simulink model "SIR"  (R2024b)
settings: Solver=VariableStepAuto  StartTime=0.0  StopTime=50.0  RelTol=1e-3
settings Model: Creator=max  LastModifiedBy=max

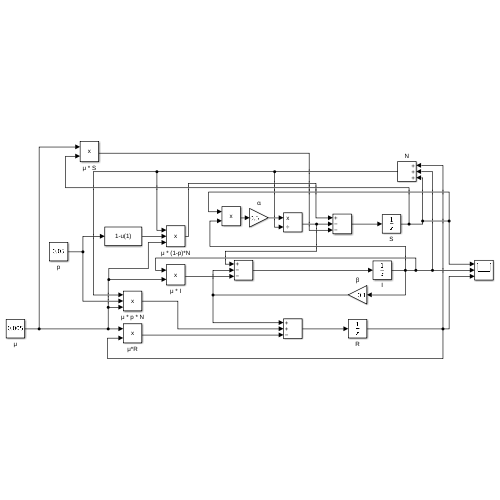
[thumbnail: Simulink's stored preview of the top-level diagram]
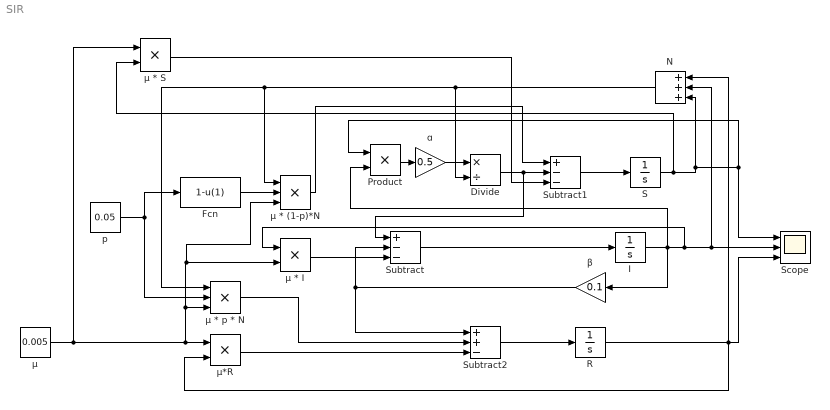
== system SIR ==
  Divide : Product  Inputs=*/
  Fcn : Fcn  Expr=1-u(1)
  I : Integrator  InitialCondition=5
  N : Sum  Inputs=+++
  Product : Product
  R : Integrator
  S : Integrator  InitialCondition=995
  Scope : Scope  NumInputPorts=3
  Subtract : Sum  Inputs=+--
  Subtract1 : Sum  Inputs=+--
  Subtract2 : Sum  Inputs=++-
  p : Constant  Value=0.05
  ɑ : Gain  Gain=0.5
  β : Gain  Gain=0.1
  μ : Constant  Value=0.005
  μ * (1-p)*N : Product  Inputs=3
  μ * I : Product
  μ * S : Product
  μ * p * N : Product  Inputs=3
  μ*R : Product
  wires:
  I/1 -> Product/2, β/1, μ * I/1, N/2, Scope/2
  R/1 -> N/1, μ*R/2, Scope/3
  β/1 -> Subtract2/1, Subtract/2
  Subtract/1 -> I/1
  S/1 -> μ * S/2, N/3, Product/1, Scope/1
  Product/1 -> ɑ/1
  ɑ/1 -> Divide/1
  N/1 -> Divide/2, μ * (1-p)*N/1, μ * p * N/1
  Divide/1 -> Subtract/1, Subtract1/2
  Subtract1/1 -> S/1
  Subtract2/1 -> R/1
  p/1 -> Fcn/1, μ * p * N/2
  μ/1 -> μ * p * N/3, μ * (1-p)*N/3, μ * I/2, μ*R/1, μ * S/1
  μ*R/1 -> Subtract2/3
  μ * p * N/1 -> Subtract2/2
  μ * I/1 -> Subtract/3
  Fcn/1 -> μ * (1-p)*N/2
  μ * (1-p)*N/1 -> Subtract1/1
  μ * S/1 -> Subtract1/3
